simulink subsystem "IMU"  (R2024b)
settings: Solver=VariableStepAuto  StartTime=0.0  StopTime=10.0  RelTol=1e-3
model mask{Ssi=[1 0 0; 0 1 0; 0 0 1], Lsi=[0 0 0], noise_pres=[0.2], noise_accel=[1 1 1]*10e-3, noise_gyro=[1 1 1]*10e-9, noise_mag=[1,1,1]*1e-2, noise_attitude_quat=[1,1,1,1]*1e-6, bias_accel=[0 0 0], scale_accel=[1 0 0; 0 1 0; 0 0 1], lim_accel=0, bias_gyro=[0.001 -0.002 -0.001], scale_gyro=[1 0 0; 0 1 0; 0 0 1], lim_gyro=0, lat=43.4643, lon=80.5204, year=2025}
  mask prompts: Ssi "Body to Sensor rotation"; Lsi "Sensor Location in Body frame"; noise_pres "Pressure Noise Power"; noise_accel "Accelerometer Noise Power"; noise_gyro "Gyro Noise Power"; noise_mag "Mag Noise Power"; noise_attitude_quat "AHRS Noise Power"; bias_accel "Accelerometer Bias"; scale_accel "Accelerometer Scaling"; lim_accel "Accelerometer Limit"; bias_gyro "Gyro Bias"; scale_gyro "Gyro Scaling"; lim_gyro "Gyro Limit"; lat "Geodetic Latitude (deg)"; lon "Geodetic Longitude (deg)"
undefined symbols (not defined in the file or in its folder): location, samplingrate
libraries: simulink x3, aerolibatmos2 x1, aerolibnav x1
settings Model: Creator=finnb  LastModifiedBy=finnb

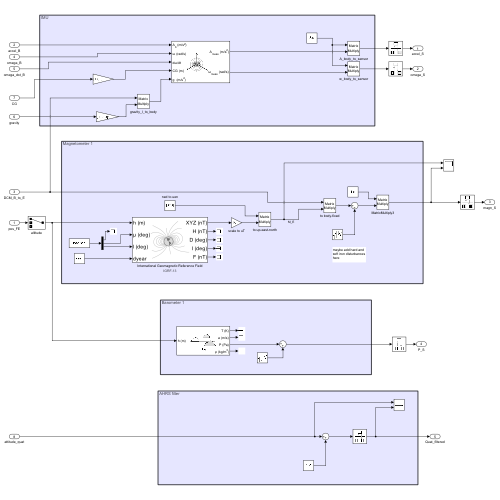
[thumbnail: Simulink's stored preview of the top-level diagram]
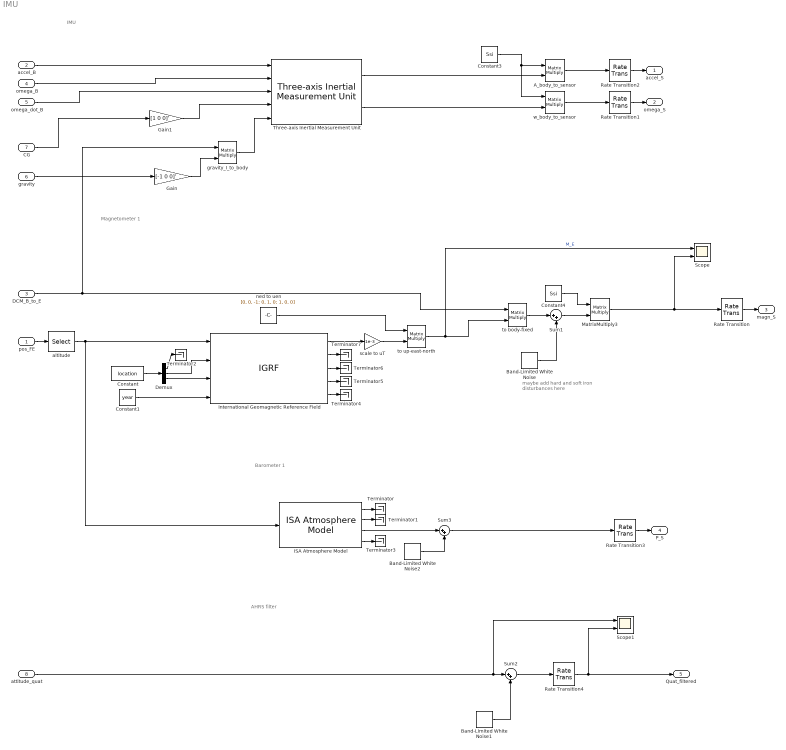
== system IMU ==
  note: AHRS filter
  note: Barometer 1
  note: Magnetometer 1
  note: IMU
  note: maybe add hard and soft iron disturbances here
  pos_FE : Inport
  accel_B : Inport  Port=2
  DCM_B_to_E : Inport  Port=3
  omega_B : Inport  Port=4
  omega_dot_B : Inport  Port=5
  gravity : Inport  Port=6
  CG : Inport  Port=7
  attitude_quat : Inport  Port=8
  A_body_to_sensor : Product  Multiplication=Matrix(*)
  Band-Limited White Noise : simulink/Sources/Band-Limited White Noise  Cov=noise_mag  Ts=samplingrate  seed=[23341]
  Band-Limited White Noise1 : simulink/Sources/Band-Limited White Noise  Cov=noise_attitude_quat  Ts=samplingrate  seed=[2323451]
  Band-Limited White Noise2 : simulink/Sources/Band-Limited White Noise  Cov=noise_pres  Ts=samplingrate  seed=[5781]
  Constant : Constant  Value=location
  Constant1 : Constant  Value=year
  Constant3 : Constant  Value=Ssi
  Constant4 : Constant  Value=Ssi
  Demux : Demux  Outputs=3
  Gain : Gain  Gain=[-1 0 0]'
  Gain1 : Gain  Gain=[1 0 0]'
  ISA Atmosphere Model : aerolibatmos2/ISA Atmosphere Model  useExtended=on  action=Warning  custom=off  viscosityOut=off  g=9.80665  gamma=1.4  R=287.0531  L=0.0065  h_trop=11000  h_strat=20000  rho0=1.225  P0=101325  T0=288.15  h0=0  S=110.4  Tref=273.15  muref=1.716e-5
  International Geomagnetic Reference Field : IGRF  month=January  day=1  year=2020  sv_out=off
      settings: AttributesFormatString=%<generation>
  MatrixMultiply3 : Product  Multiplication=Matrix(*)
  Rate Transition{,1..4} (5 alike) : RateTransition  OutPortSampleTime=samplingrate
  Scope : Scope  NumInputPorts=2
  Scope1 : Scope  NumInputPorts=2
  Sum1 : Sum  Inputs=|++
  Sum2 : Sum  Inputs=|++
  Sum3 : Sum  Inputs=|++
  Terminator{,1..7} (8 alike) : Terminator
  Three-axis Inertial Measurement Unit : aerolibnav/Three-axis Inertial Measurement Unit  units=Metric (MKS)  imu=Lsi  i_Ts=samplingrate  dtype_a=off  w_a=190  z_a=0.707  a_sf_cc=scale_accel  a_bias=bias_accel  a_sat="[-lim_accel  -lim_accel  -lim_accel  lim_accel lim_accel lim_accel]"  dtype_g=off  w_g=190  z_g=0.707  g_sf_cc=scale_gyro  g_bias=bias_gyro  g_sens=[0 0 0]  g_sat="[-lim_gyro  -lim_gyro  -lim_gyro lim_gyro lim_gyro lim_gyro]"  i_rand=on  i_seeds=[23093 23094 23095 23096 23097 23098]  i_pow="[noise_accel,  noise_gyro]"
  altitude : Selector  InputPortWidth=3  IndexOptions=Index vector (dialog)  Indices=[1]  OutputSizes=1
  gravity_I_to_body : Product  Multiplication=Matrix(*)
  ned to uen : Constant  Value=[0, 0, -1; 0, 1, 0; 1, 0, 0]
  scale to uT : Gain  Gain=1e-3
  to body-fixed : Product  Multiplication=Matrix(*)
  to up-east-north : Product  Multiplication=Matrix(*)
  w_body_to_sensor : Product  Multiplication=Matrix(*)
  accel_S : Outport
  omega_S : Outport  Port=2
  magn_S : Outport  Port=3
  P_S : Outport  Port=4
  Quat_filtered : Outport  Port=5
  wires:
  accel_B/1 -> Three-axis Inertial Measurement Unit/1
  omega_B/1 -> Three-axis Inertial Measurement Unit/2
  omega_dot_B/1 -> Three-axis Inertial Measurement Unit/3
  CG/1 -> Gain1/1
  gravity_I_to_body/1 -> Three-axis Inertial Measurement Unit/5
  Gain1/1 -> Three-axis Inertial Measurement Unit/4
  Constant/1 -> Demux/1
  Demux/2 -> International Geomagnetic Reference Field/2
  International Geomagnetic Reference Field/1 -> scale to uT/1
  to up-east-north/1 -> to body-fixed/2, Scope/1  "M_E"
  Band-Limited White Noise/1 -> Sum1/2
  Rate Transition/1 -> magn_S/1
  Sum1/1 -> MatrixMultiply3/2
  Rate Transition1/1 -> omega_S/1
  Rate Transition2/1 -> accel_S/1
  A_body_to_sensor/1 -> Rate Transition2/1
  Constant3/1 -> w_body_to_sensor/1, A_body_to_sensor/1
  w_body_to_sensor/1 -> Rate Transition1/1
  Sum3/1 -> Rate Transition3/1
  ISA Atmosphere Model/3 -> Sum3/1
  Band-Limited White Noise2/1 -> Sum3/2
  Constant4/1 -> MatrixMultiply3/1
  Rate Transition3/1 -> P_S/1
  Gain/1 -> gravity_I_to_body/2
  gravity/1 -> Gain/1
  Demux/3 -> International Geomagnetic Reference Field/3
  pos_FE/1 -> altitude/1
  Demux/1 -> Terminator2/1
  altitude/1 -> ISA Atmosphere Model/1, International Geomagnetic Reference Field/1
  Constant1/1 -> International Geomagnetic Reference Field/4
  to body-fixed/1 -> Sum1/1
  ned to uen/1 -> to up-east-north/1
  scale to uT/1 -> to up-east-north/2
  DCM_B_to_E/1 -> to body-fixed/1, gravity_I_to_body/1
  Three-axis Inertial Measurement Unit/1 -> A_body_to_sensor/2
  Three-axis Inertial Measurement Unit/2 -> w_body_to_sensor/2
  MatrixMultiply3/1 -> Rate Transition/1, Scope/2
  ISA Atmosphere Model/1 -> Terminator/1
  ISA Atmosphere Model/2 -> Terminator1/1
  ISA Atmosphere Model/4 -> Terminator3/1
  International Geomagnetic Reference Field/5 -> Terminator4/1
  International Geomagnetic Reference Field/4 -> Terminator5/1
  International Geomagnetic Reference Field/3 -> Terminator6/1
  International Geomagnetic Reference Field/2 -> Terminator7/1
  Band-Limited White Noise1/1 -> Sum2/2
  Rate Transition4/1 -> Scope1/2, Quat_filtered/1
  Sum2/1 -> Rate Transition4/1
  attitude_quat/1 -> Scope1/1, Sum2/1
